simulink model "NonLinModelMracScaled"  (R2023b)
settings: Solver=ode4  StartTime=0.0  StopTime=150  FixedStep=1e-4  RelTol=1e-3
values from neighbouring files (symbols this model uses):
  AEFF = 2.0106e-04    (= 0.00020106)    [apply_itsmrac.m]    (also in mrac_debug_05Hz.m; mrac_final_solution.m; mrac_fix_and_sweep.m; optimize_mrac.m)
  Am_bar = A_bar - B_bar_mA * Km    [apply_itsmrac.m]    (also in mrac_debug_05Hz.m; mrac_final_solution.m; mrac_fix_and_sweep.m; optimize_mrac.m)
  B_E = 1.6e9    (= 1600000000)    [apply_itsmrac.m]    (also in mrac_debug_05Hz.m; mrac_final_solution.m; mrac_fix_and_sweep.m; optimize_mrac.m)
  Bm_bar_mm = B_bar_mA / DC_gain    [apply_itsmrac.m]    (also in mrac_debug_05Hz.m; mrac_final_solution.m; mrac_fix_and_sweep.m; optimize_mrac.m)
  C_T = 3.9933e-13    [apply_itsmrac.m]    (also in mrac_debug_05Hz.m; mrac_final_solution.m; mrac_fix_and_sweep.m; optimize_mrac.m)
  Gamma_L = 1e-6    (= 1e-06)    [apply_itsmrac.m]    (also in mrac_debug_05Hz.m = 1e-10; mrac_final_solution.m = 1e-10; mrac_fix_and_sweep.m = 1e-11; newDesign.m)
  Gamma_R = 1e-5    (= 1e-05)    [apply_itsmrac.m]    (also in mrac_debug_05Hz.m = 1e-09; mrac_final_solution.m = 1e-09; mrac_fix_and_sweep.m = 1e-10; newDesign.m)
  k = 1.82709080    (= 1.8270908)    [apply_itsmrac.m]    (also in mrac_debug_05Hz.m; mrac_final_solution.m; mrac_fix_and_sweep.m; optimize_mrac.m)
  K = 0.00000334    (= 3.34e-06)    [apply_itsmrac.m]    (also in mrac_debug_05Hz.m; mrac_final_solution.m; mrac_fix_and_sweep.m; optimize_mrac.m)
  L_hat_IC = -Km    [apply_itsmrac.m]    (also in mrac_debug_05Hz.m; mrac_final_solution.m; mrac_fix_and_sweep.m; newDesign.m)
  M = 3.4    [apply_itsmrac.m]    (also in mrac_debug_05Hz.m = M(1:len); mrac_final_solution.m; mrac_fix_and_sweep.m; optimize_mrac.m)
  m3PsToLpm = 60e3    (= 60000)    [apply_itsmrac.m]    (also in mrac_debug_05Hz.m; mrac_final_solution.m; mrac_fix_and_sweep.m; optimize_mrac.m)
  M_hat_IC = 1 / DC_gain    [apply_itsmrac.m]    (also in mrac_debug_05Hz.m; mrac_final_solution.m; mrac_fix_and_sweep.m; newDesign.m)
  P_bar = lyap(Am_bar', eye(3))    [apply_itsmrac.m]    (also in mrac_debug_05Hz.m; mrac_final_solution.m; mrac_fix_and_sweep.m; newDesign.m = lyap(Am_bar', Q_bar))
  P_return = 4.46e5    (= 446000)    [apply_itsmrac.m]    (also in mrac_debug_05Hz.m; mrac_final_solution.m; mrac_fix_and_sweep.m; newDesign.m)
  PA_IC = Ps_supply/2    (= 9992500)    [apply_itsmrac.m]    (also in mrac_debug_05Hz.m; mrac_final_solution.m; mrac_fix_and_sweep.m; newDesign.m = PA_Pa.Data(1))
  PB_IC = Ps_supply/2    (= 9992500)    [apply_itsmrac.m]    (also in mrac_debug_05Hz.m; mrac_final_solution.m; mrac_fix_and_sweep.m; newDesign.m = PB_Pa.Data(1))
  PB_vec = [P_bar(1,:) * B_bar_mA; 0; 0]    [apply_itsmrac.m]    (also in mrac_debug_05Hz.m; mrac_final_solution.m; mrac_fix_and_sweep.m = P_bar * B_bar_mA; optimize_mrac.m)
  Ps_supply = 199.85e5    (= 19985000)    [apply_itsmrac.m]    (also in mrac_debug_05Hz.m; mrac_final_solution.m; mrac_fix_and_sweep.m; newDesign.m)
  sigma_L = 0.001    [apply_itsmrac.m]    (also in mrac_debug_05Hz.m = 0.01; mrac_final_solution.m = 0.05; mrac_fix_and_sweep.m = 0.01; newDesign.m)
  sigma_M = 0.001    [apply_itsmrac.m]    (also in mrac_debug_05Hz.m = 0.01; mrac_final_solution.m = 0.05; mrac_fix_and_sweep.m = 0.01; newDesign.m)
  V01 = AEFF * (L_STROKE/2)    (= 1.91167848e-05)    [apply_itsmrac.m]    (also in mrac_debug_05Hz.m; mrac_final_solution.m; mrac_fix_and_sweep.m; optimize_mrac.m)
  V02 = V01    (= 1.91167848e-05)    [apply_itsmrac.m]    (also in mrac_debug_05Hz.m; mrac_final_solution.m; mrac_fix_and_sweep.m; optimize_mrac.m)
  V_DEAD = 1.5315e-05    [apply_itsmrac.m]    (also in mrac_debug_05Hz.m; mrac_final_solution.m; mrac_fix_and_sweep.m; optimize_mrac.m)
  xc_dot_IC = v_mPs.Data(1)    [newDesign.m]
  xc_IC = xc_m.Data(1)    [newDesign.m]
undefined symbols (not defined in the file or in its folder): PA_Pa, PB_Pa, r_v_mPs, xc_m
(part 2 of 2)

== matlab function NonLinModelMracScaled/Plant/Cylinder_Dynamics/MATLAB Function1 ==
  data: v input; FF output; a input; j input
function FF = fcn(v,a,j)
% --- Geçiş Yumuşaklığı Parametresi ---
% Bu değer büyüdükçe 0'daki eğim azalır (daha eğimli geçer)
eps_smooth = 0.00223;


% --- Pozitif Yön (v > 0) ---
kv_p = 39.658; Fc_p = 25; Fs_p = 82.9; tau_p = 0.0016;

% --- Negatif Yön (v < 0) ---
kv_n = 38.5; Fc_n = 5; Fs_n = 75.17; tau_n = 0.0016;

% Yumuşatılmış yön fonksiyonu (sign yerine tanh)
% Bu fonksiyon -1 ile 1 arasında yumuşak bir geçiş sağlar
smooth_sign = tanh(v ./ eps_smooth);

% Asimetrik katsayı vektörleri oluşturma
% Hızın yönüne göre katsayıları seçiyoruz
kv = (v >= 0)*kv_p + (v < 0)*kv_n;
Fc = (v >= 0)*Fc_p + (v < 0)*Fc_n;
Fs = (v >= 0)*Fs_p + (v < 0)*Fs_n;
tau = (v >= 0)*tau_p + (v < 0)*tau_n;

F_stribeck = (kv .* v) + (Fc .* smooth_sign) + (Fs .* smooth_sign .* exp(-abs(v./tau)));

K_acc = 1.121235; 
K_jerk = 0.056481; 
kappa_delay = 0; 

FF = F_stribeck + K_acc * a  +  K_jerk*j;
